simulink model "Es2_l7_simulink"  (R2024b)
settings: Solver=ode45  StartTime=0.0  StopTime=t_sim  MaxStep=0.001*Ts  MinStep=0.0001*Ts  RelTol=1e-3
values from neighbouring files (symbols this model uses):
  d1 = 0    [Es2_l7.m]
  d2 = 0    [Es2_l7.m]
  rho = 1    [Es2_l7.m]
  Ts = 0.005    [Es2_l7.m]    (also in Lab_Practice7_2.m)
undefined symbols (not defined in the file or in its folder): DiscIntNeverNeededParam
libraries: cstblocks x2, simulink x2
settings Model: Creator=Claudio Calabrese  LastModifiedBy=Claudio Calabrese
settings SolverCC: InitialStep=0.0001*Ts

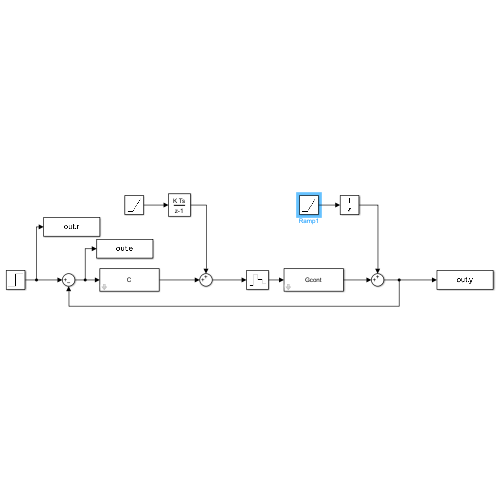
[thumbnail: Simulink's stored preview of the top-level diagram]
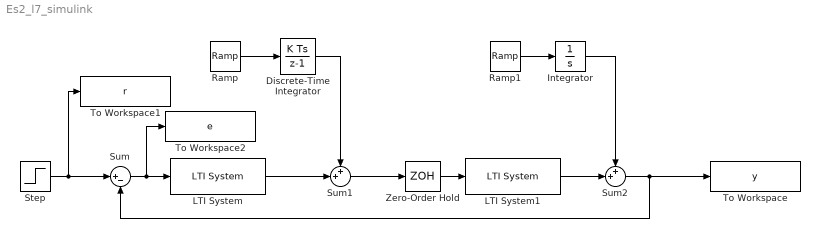
== system Es2_l7_simulink ==
  Discrete-Time Integrator : DiscreteIntegrator  SampleTime=Ts  ICPrevOutput=DiscIntNeverNeededParam  ICPrevScaledInput=DiscIntNeverNeededParam
  Integrator : Integrator
  LTI System : cstblocks/LTI System  sys=C  IC=[]  PadeOrder=0
  LTI System1 : cstblocks/LTI System  sys=Gcont  IC=[]  PadeOrder=0
  Ramp : simulink/Sources/Ramp  slope=d1  start=0  InitialOutput=0
  Ramp1 : simulink/Sources/Ramp  slope=d2  start=0  InitialOutput=0
  Step : Step  Time=0  After=rho  SampleTime=Ts
  Sum : Sum  Inputs=|+-
  Sum1 : Sum  Inputs=++|
  Sum2 : Sum  Inputs=++|
  To Workspace : ToWorkspace  VariableName=y  SaveFormat=Timeseries  SampleTime=Ts
  To Workspace1 : ToWorkspace  VariableName=r  SaveFormat=Timeseries  SampleTime=Ts
  To Workspace2 : ToWorkspace  VariableName=e  SaveFormat=Timeseries  SampleTime=Ts
  Zero-Order Hold : ZeroOrderHold  SampleTime=Ts
  wires:
  Step/1 -> To Workspace1/1, Sum/1
  Sum/1 -> To Workspace2/1, LTI System/1
  LTI System/1 -> Sum1/2
  Sum1/1 -> Zero-Order Hold/1
  Zero-Order Hold/1 -> LTI System1/1
  LTI System1/1 -> Sum2/2
  Sum2/1 -> To Workspace/1, Sum/2
  Ramp/1 -> Discrete-Time Integrator/1
  Discrete-Time Integrator/1 -> Sum1/1
  Ramp1/1 -> Integrator/1
  Integrator/1 -> Sum2/1
